simulink model "Rule_based_stop_if_likely_collision_simulink_joystick_from_odom"  (R2023a)
settings: Solver=FixedStepAuto  StartTime=0.0  StopTime=inf  RelTol=1e-3
model workspace (MAT data in the model file):
  SL_ROS_VariableLengthArrays_MaxSizes.CommonInfo.ArrayTruncateAction = 'EmitWarning'
  SL_ROS_VariableLengthArrays_MaxSizes.MsgTypeMap = containers.Map
  SL_ROS_VariableLengthArrays_MaxSizes.MsgTypeMap.serialization.keys = {'sensor_msgs/LaserScan'}
  SL_ROS_VariableLengthArrays_MaxSizes.MsgTypeMap.serialization.values{1}(1).PropertyName = 'intensities'
  SL_ROS_VariableLengthArrays_MaxSizes.MsgTypeMap.serialization.values{1}(1).DataType = 'single'
  SL_ROS_VariableLengthArrays_MaxSizes.MsgTypeMap.serialization.values{1}(1).MaxLength = 360
  SL_ROS_VariableLengthArrays_MaxSizes.MsgTypeMap.serialization.values{1}(2).PropertyName = 'ranges'
  SL_ROS_VariableLengthArrays_MaxSizes.MsgTypeMap.serialization.values{1}(2).DataType = 'single'
  SL_ROS_VariableLengthArrays_MaxSizes.MsgTypeMap.serialization.values{1}(2).MaxLength = 360
  SL_ROS_VariableLengthArrays_MaxSizes.MsgTypeMap.serialization.uniformity = 0
  SL_ROS_VariableLengthArrays_MaxSizes.MsgTypeMap.serialization.keyType = 'char'
  SL_ROS_VariableLengthArrays_MaxSizes.MsgTypeMap.serialization.valueType = 'any'
values from neighbouring files (symbols this model uses):
  scan = lidarScan(ranges,angles)    [rule_based_obstacles_avoidance_stop_if_likely_collision.m]
undefined symbols (not defined in the file or in its folder): angular, linear
libraries: ros2lib x5, vrlib x1
settings Model: Creator=fede  LastModifiedBy=fede
settings OptimizationCC: EnhancedBackFolding=on  PassReuseOutputArgsAs=Individual arguments  ZeroExternalMemoryAtStartup=off  ZeroInternalMemoryAtStartup=off  MaxStackSize=64  OptimizeBlockOrder=speed  DifferentSizesBufferReuse=on  OptimizationCustomize=off  EfficientTunableParamExpr=on
settings DebuggingCC: ParameterTunabilityLossMsg=error
settings HardwareCC: ProdBitPerLong=64  ProdHWDeviceType=Intel->x86-64 (Linux 64)  UseEmbeddedCoderFeatures=off
settings SFSimCC: MATLABDynamicMemAlloc=off
settings RTWCC: Description=Embedded Coder  SystemTargetFile=ert.tlc  HardwareBoard=Robot Operating System 2 (ROS 2)  TLCOptions="-aInlineSetEventsForThisBaseRateFcn=TLC_FALSE -aSuppressMultiTaskScheduler=TLC_FALSE  -aRateBasedStepFcn=0"  TemplateMakefile=ert_default_tmf  Toolchain=Colcon Tools  TargetLang=C++
settings CodeAppCC: ForceParamTrailComments=on  IgnoreCustomStorageClasses=off  OperatorAnnotations=on  SimulinkDataObjDesc=on  SFDataObjDesc=on  InsertBlockDesc=on
settings ERTTargetCC: CodeInterfacePackaging=C++ class  SupportNonInlinedSFcns=on  RootIOFormat=Structure reference

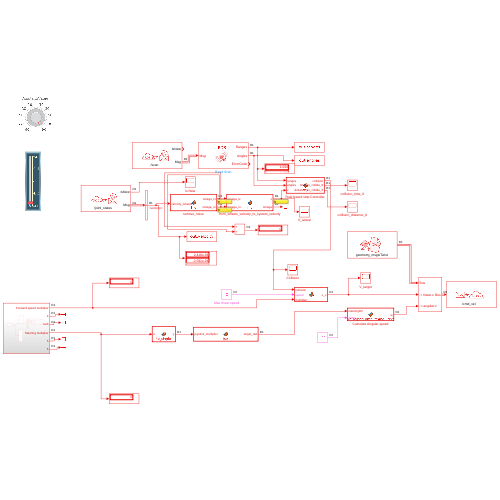
[thumbnail: Simulink's stored preview of the top-level diagram]
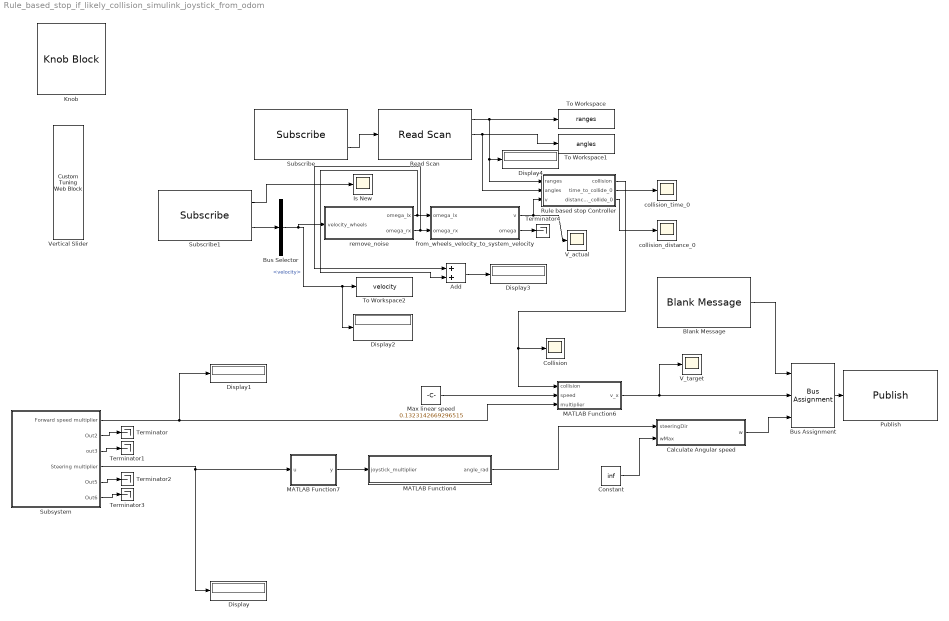
== system Rule_based_stop_if_likely_collision_simulink_joystick_from_odom ==
  Add : Sum
  Blank Message : ros2lib/Blank Message  messageClass=Message  entityType=geometry_msgs/Twist  messageType=geometry_msgs/Twist  SampleTime=0.01
  Bus Assignment : BusAssignment  AssignedSignals=linear.x,angular.z
  Bus Selector : BusSelector  OutputSignals=velocity
  Calculate Angular speed : MATLAB Function  TreatAsAtomicUnit=on
  Collision : Scope
  Constant : Constant  Value=inf
  Display{,1..4} (5 alike) : Display
  Is New : Scope
  Knob : KnobBlock  ScaleMin=-90  ScaleMax=90
  MATLAB Function4 : MATLAB Function  TreatAsAtomicUnit=on  SystemSampleTime=0.01
  MATLAB Function6 : MATLAB Function  TreatAsAtomicUnit=on  SystemSampleTime=0.01
  MATLAB Function7 : MATLAB Function  TreatAsAtomicUnit=on
  Max linear speed : Constant  Value=0.1323142669296515
  Publish : ros2lib/Publish  topicSource=Select from ROS network  topic=/cmd_vel  messageType=geometry_msgs/Twist  QOSHistory=Keep last  QOSDepth=1  QOSReliability=Reliable  QOSDurability=Volatile
  Read Scan : ros2lib/Read Scan  MaximumArrayLength=180  ShowAnglesOutput=on  ShowIntensityOutput=off  ShowErrorCodeOutput=on  VariableSizeOutputs=off
  Rule based stop Controller : MATLAB Function  TreatAsAtomicUnit=on
  Subscribe : ros2lib/Subscribe  topicSource=Select from ROS network  topic=/scan  messageType=sensor_msgs/LaserScan  sampleTime=0.01  QOSHistory=Keep last  QOSDepth=1  QOSReliability=Reliable  QOSDurability=Volatile
  Subscribe1 : ros2lib/Subscribe  topicSource=Select from ROS network  topic=/joint_states  messageType=sensor_msgs/JointState  sampleTime=0.01  QOSHistory=Keep last  QOSDepth=1  QOSReliability=Reliable  QOSDurability=Volatile
  Subsystem : Subsystem
  Terminator{,1..4} (5 alike) : Terminator
  To Workspace : ToWorkspace  VariableName=ranges  SaveFormat=Timeseries  SampleTime=-1
  To Workspace1 : ToWorkspace  VariableName=angles  SaveFormat=Timeseries  SampleTime=-1
  To Workspace2 : ToWorkspace  VariableName=velocity  SaveFormat=Timeseries  SampleTime=-1
  V_actual : Scope
  V_target : Scope
  Vertical Slider : CustomTuningWebBlock  LabelPosition=Hide  ShowInitialText=on  Configuration="{\"components\":[{\"name\":\"LinearScaleComponent\",\"settings\":{\"bounds\":{\"max\":2,\"min\":0,\"tickInterval\":\"auto\"},\"internalTickHeightScaleFactor\":0.5,\"labelColor\":[255,255,200],\"labelFont\":{\"font\":\"Arial\",\"fontSize\":12},\"labelOffset\":0.05,\"labelTransparency\":1,\"needleImage\":{\"size\":[596,842],\"src\":\"data:image\\/svg+xml;base64,PD94bWwgdmVyc2lvbj0iMS4wIiBlbmNvZGluZz0idXRmLTgiPz4NCjwhLS0gR2VuZXJhdG9yOiBBZG9iZSBJbGx1c3RyYXRvciAyNS4wLjAsIFNWRyBFeHBvcnQgUGx1Zy1JbiAuIFNWRyBWZXJzaW9uOiA2LjAwIEJ1aWxkIDApICAtLT4NCjxzdmcgdmVyc2lvbj0iMS4xIg0KCSBpZD0ic3ZnOCIgeG1sbnM6Y2M9Imh0dHA6Ly9jcmVhdGl2ZWNvbW1vbnMub3JnL25zIyIgeG1sbnM6ZGM9Imh0dHA6Ly9wdXJsLm9yZy9kYy9lbGVtZW50cy8xLjEvIiB4bWxuczppbmtzY2FwZT0iaHR0cDovL3d3dy5pbmtzY2FwZS5vcmcvbmFtZXNw ...(+2420 chars)\",\"srcOrientation\":\"horizontal\"},\"needleOffset\":[0.0642123287671233,-0.8044596912521441],\"needleSize\":{\"height\":0.07668067226890757,\"width\":0.4337797619047619},\"position\":[0.03623949579831933,0.2829861111111111,0.6088789682539683,0.9196428571428571],\"referencePoint\":\"auto\",\"scaleColors\":[],\"scaleColorsSize\":0.2,\"scaleDirection\":\"BT\",\"showLabels\":1,\"showMinorTicks\":0,\"showSpanLine\":1,\"showTicks\":1,\"tickColor\":[252,252,197],\"tickTransparency\":1,\"valueBarColor\":[0,114,189],\"valueBarOffset\":-0.27,\"valueBarSize\":0.1,\"valueBarTransparency\":1}},{\"name\":\"BackgroundImageComponent\",\"settings\":{\"image\":{\"size\":[380,101],\"src\":\"data:image\\/svg+xml;base64,PHN2ZyB4bWxucz0iaHR0cDovL3d3dy53My5vcmcvMjAwMC9zdmciIHhtbG5zOnhsaW5rPSJodHRwOi8vd3d3LnczLm9yZy8xOTk5L3hsaW5rIiB2aWV3Qm94PSIwIDAgMzgwIDEwMSI+PGRlZnM+PHN0eWxlPi5jbHMtMXtmaWxsOiMwMDJiNDI7fS5jbHMtMntmaWxsOiM0MjcwODI7fS5jbHMtM3tmaWxsOnVybCgjcmFkaWFsLWdyYWRpZW50KTt9LmNscy00e2ZpbGw6I2M4YzhjODtzdHJva2U6IzAwMDt9PC9zdHlsZT48cmFkaWFsR3JhZGllbnQgaWQ9InJhZGlhbC1ncmFkaWVudCIgY3g9IjE5MCIgY3k9IjUwLjUiIHI9IjI2OS4yMSIgZ3JhZGllbnRVbml0cz0idXNlclNwYWNlT25Vc2UiPjxzdG9wIG9mZnNldD0iMC4wMSIgc3RvcC1jb2xvcj0iIzNlNGY1OCIvPjxzdG9wIG9mZnNldD0iMC4wNiIgc3RvcC1jb2xvcj0iIzQ0NTc2MSIvPjxzdG9wIG9mZnNldD0iMC4xNSIgc3RvcC1jb2xvcj0iIzU1NmE3NiIvPjxzdG9wIG9mZnNldD0iMC4yNSIgc3RvcC1jb2xvcj0iIzZkODg5NSIvPjxzdG9wIG9mZnNldD0iMC4zOCIgc3RvcC1jb2xvcj0iIzhmYjJjMyIvPjxzdG9wIG9mZnNldD0iMC41MiIgc3RvcC1jb2xvcj0iI2I2ZTRmYSIvPjxzdG9wIG9mZnNldD0iMSIgc3RvcC1jb2xvcj0iIzE1NDY1NyIvPjwvcmFkaWFsR3JhZGllbnQ+PC9kZWZzPjxnIGlkPSJmcmFtZSI+PGcgaWQ9IkxheWVyXzIiIGRhdGEtbmFtZT0iTGF5ZXIgMiI+PGcgaWQ9IkxheWVyXzEtMiIgZGF0YS1uYW1lPSJMYXllciAxLTIiPjxyZWN0IGlkPSJyZWN0MTAzNiIgY2xhc3M9ImNscy0xIiB4PSIxMSIgeT0iMTEiIHdpZHRoPSIzNTgiIGhlaWdodD0iNzkiLz48cGF0aCBpZD0icGF0aDEwMzgiIGNsYXNzPSJjbHMtMiIgZD0iTTgsOFY5M0gzNzJWOFpNMzY5LDkwSDExVjExSDM2OVoiLz48cGF0aCBpZD0icGF0aDEwNDAiIGNsYXNzPSJjbHMtMyIgZD0iTTAsMFYxMDFIMzgwVjBaTTM3Miw5M0g4VjhIMzcyWiIvPjwvZz48L2c+PC9nPjxnIGlkPSJ0cmFjayI+PHBhdGggaWQ9InJlY3QxNjExIiBjbGFzcz0iY2xzLTQiIGQ9Ik0zMy4zNywyNi41OUgzNDYuNjNjNCwwLDcuMjUsMi42LDcuMjUsNS44MWgwYzAsMy4yMS0zLjI1LDUuODItNy4yNSw1LjgySDMzLjM3Yy00LDAtNy4yNS0yLjYxLTcuMjUtNS44MmgwQzI2LjEyLDI5LjE5LDI5LjM3LDI2LjU5LDMzLjM3LDI2LjU5WiIvPjwvZz48L3N2Zz4=\",\"srcOrientation\":\"horizontal\"},\"position\":[0,0,1,1],\"scaleMode\":\"0\"}},{\"name\":\"ForegroundImageComponent\",\"settings\":{\"image\":{\"size\":[0,0],\"src\":\"default\",\"srcOrientation\":[]},\"isForeground\":1,\"position\":[0,0,1,1],\"scaleMode\":\"0\"}}],\"settings\":{\"BindingType\":\"param\",\"aspectRatio\":3.7777777777777777,\"backgroundColor\":[0,0,0,\"1\"],\"backgroundOffset\":0,\"backgroundOpacity\":1,\"fixedAspectRatio\":\"on\",\"foregroundColor\":[252,252,196],\"orientation\":\"vertical\",\"showBackgroundColor\":false,\"value\":0,\"version\":\"R2023a\"},\"type\":\"LinearGauge\"}"
  collision_distance_0 : Scope
  collision_time_0 : Scope
  from_wheels_velocity_to_system_velocity : MATLAB Function  TreatAsAtomicUnit=on  SystemSampleTime=0.01
  remove_noise : MATLAB Function  TreatAsAtomicUnit=on  SystemSampleTime=0.01
  wires:
  Subscribe/2 -> Read Scan/1
  Read Scan/2 -> To Workspace1/1, Rule based stop Controller/2(angles)
  Blank Message/1 -> Bus Assignment/1
  Bus Assignment/1 -> Publish/1
  Subsystem/3(out3) -> Terminator1/1
  Subsystem/5(Out5) -> Terminator2/1
  Subsystem/6(Out6) -> Terminator3/1
  Subsystem/2(Out2) -> Terminator/1
  MATLAB Function6/1(v_x) -> V_target/1, Bus Assignment/2
  Max linear speed/1 -> MATLAB Function6/2(speed)
  MATLAB Function7/1(y) -> MATLAB Function4/1(joystick_multiplier)
  Calculate Angular speed/1(w) -> Bus Assignment/3
  Constant/1 -> Calculate Angular speed/2(wMax)
  Bus Selector/1 -> remove_noise/1(velocity_wheels), To Workspace2/1, Display2/1  "<velocity>"
  Rule based stop Controller/1(collision) -> Collision/1, MATLAB Function6/1(collision)
  MATLAB Function4/1(angle_rad) -> Calculate Angular speed/1(steeringDir)
  Subsystem/4(Steering multiplier) -> Display/1, MATLAB Function7/1(u)
  Subsystem/1(Forward speed multiplier) -> Display1/1, MATLAB Function6/3(multiplier)
  Subscribe1/2 -> Bus Selector/1
  Subscribe1/1 -> Is New/1
  from_wheels_velocity_to_system_velocity/1(v) -> Rule based stop Controller/3(v), V_actual/1
  from_wheels_velocity_to_system_velocity/2(omega) -> Terminator4/1
  remove_noise/1(omega_lx) -> Add/2, from_wheels_velocity_to_system_velocity/1(omega_lx)
  remove_noise/2(omega_rx) -> Add/1, from_wheels_velocity_to_system_velocity/2(omega_rx)
  Add/1 -> Display3/1
  Read Scan/1 -> To Workspace/1, Display4/1, Rule based stop Controller/1(ranges)
  Rule based stop Controller/2(time_to_collide_0) -> collision_time_0/1
  Rule based stop Controller/3(distance_to_collide_0) -> collision_distance_0/1

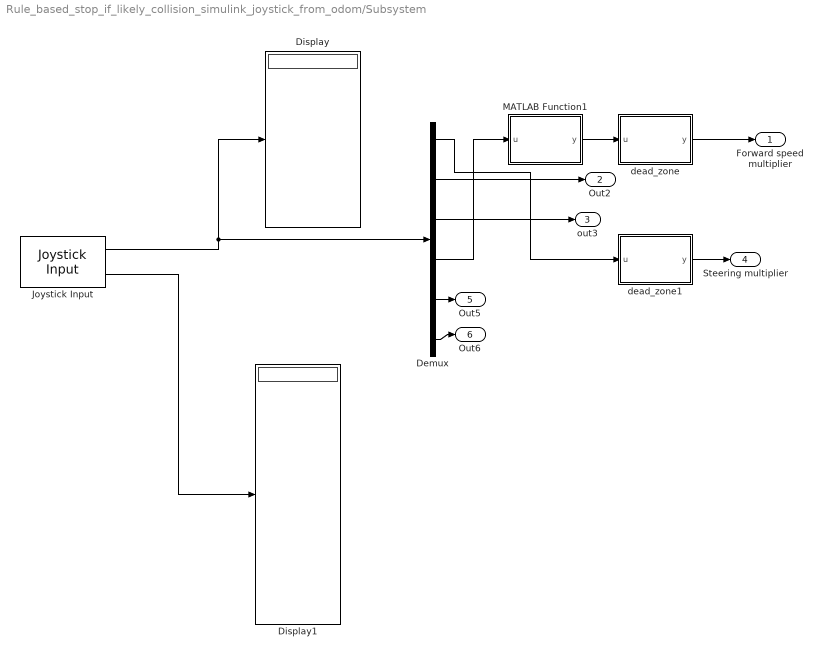
== system Rule_based_stop_if_likely_collision_simulink_joystick_from_odom/Subsystem ==
  Demux : Demux  Outputs=6
  Display : Display
  Display1 : Display
  Joystick Input : vrlib/Joystick Input  joyid=1  adjustports=on  forcefeed=off
  MATLAB Function1 : MATLAB Function  TreatAsAtomicUnit=on
  dead_zone : MATLAB Function  TreatAsAtomicUnit=on
  dead_zone1 : MATLAB Function  TreatAsAtomicUnit=on
  Forward speed multiplier : Outport
  Out2 : Outport  Port=2
  out3 : Outport  Port=3
  Steering multiplier : Outport  Port=4
  Out5 : Outport  Port=5
  Out6 : Outport  Port=6
  wires:
  Demux/2 -> Out2/1
  Demux/6 -> Out6/1
  Joystick Input/2 -> Display1/1
  Demux/5 -> Out5/1
  Joystick Input/1 -> Display/1, Demux/1
  Demux/3 -> out3/1
  MATLAB Function1/1(y) -> dead_zone/1(u)
  dead_zone/1(y) -> Forward speed multiplier/1
  dead_zone1/1(y) -> Steering multiplier/1
  Demux/4 -> MATLAB Function1/1(u)
  Demux/1 -> dead_zone1/1(u)

== matlab function Rule_based_stop_if_likely_collision_simulink_joystick_from_odom/Subsystem/MATLAB Function1 ==
  data: u input; y output
function y = fcn(u)
centered_value = u + 0.3616;

output_end = 1;
output_start = -1;
input_end = 0.7549;
input_start = -0.6384;

slope = (output_end - output_start) / (input_end - input_start);

y = -1*(output_start + slope * (centered_value - input_start));

== matlab function Rule_based_stop_if_likely_collision_simulink_joystick_from_odom/Rule based stop Controller ==
  data: ranges input; collision output; angles input; v input; time_to_collide_0 output; distance_to_collide_0 output
function [collision, time_to_collide_0, distance_to_collide_0] = fcn(ranges, angles, v)

    %Ranges, angles -> from lidar
    % v -> current wheelchair linear speed
    %Config parameters
    semi_amplitude_collision_cone_degree = 4;
    t_second_reaction_time_threshold = 3;
    %--------------

    collision_cone_rad = deg2rad(semi_amplitude_collision_cone_degree);

    %Get matrix with all 0s except 1 for elements related to the collision cone
    collision_cone_matrix_indexes = angles >= -collision_cone_rad & angles <= collision_cone_rad;
    
    %Get distances of points detected by lidar in collision cone amplitude
    collision_cone_distances = ranges(collision_cone_matrix_indexes);

    distance_to_collide_0 = collision_cone_distances(4);
    time_to_collide_0 = collision_cone_distances(4)/v;
    %Set the variable to a non-zero value if there is at least one point that is probable to collide
    %find(X,n) returns the first n indices corresponding to the nonzero elements in X.

    % Pseudo-code
    % for elem in collision_cone_distances:
    %     t = elem/v
    %     if(t<t_second_reaction_time_threshold)
    %         collision!
    if( ( v == 0 ) || ( isempty( find(collision_cone_distances/v <= t_second_reaction_time_threshold, 1) ) ) )

        collision = 0;

    elseif (v < 0) 
        % For now we decide not to take action, i.e when driving backwars
        % there is not safety system on
        collision = 0;

    else

        collision = 1;

    end

== matlab function Rule_based_stop_if_likely_collision_simulink_joystick_from_odom/Subsystem/dead_zone ==
  data: u input; y output
function y = dead_zone(u)

if(abs(u) < 0.1)
    u=0;
end

y = u;

== matlab function Rule_based_stop_if_likely_collision_simulink_joystick_from_odom/Subsystem/dead_zone1 ==
  data: u input; y output
function y = dead_zone(u)

if(abs(u) < 0.1)
    u=0;
end

y = u;

== matlab function Rule_based_stop_if_likely_collision_simulink_joystick_from_odom/from_wheels_velocity_to_system_velocity ==
  data: omega_lx input; v output double; omega output; omega_rx input
function [v,omega] = fnc(omega_lx, omega_rx)

noise_threshold = 10^-3; % obtained observing noise values

%Params
r = 0.033; %wheels radius [m]
L_r = 0.16; %distance between wheels [m]
%%%%%%%%%%%%%%%%%%%%%
v = (r / 2) * (omega_rx + omega_lx); % [m/s]

omega = (r / L_r) * (omega_rx - omega_lx); % [rad/s]

%Removing noise
if(abs(v) < noise_threshold)
    v = 0;
end

if(abs(omega) < noise_threshold)
    omega = 0;
end

== matlab function Rule_based_stop_if_likely_collision_simulink_joystick_from_odom/MATLAB Function4 ==
  data: joystick_multiplier input; angle_rad output double
function angle_rad = fcn(joystick_multiplier)

angle_rad = double(-pi/4 * joystick_multiplier);

== matlab function Rule_based_stop_if_likely_collision_simulink_joystick_from_odom/remove_noise ==
  data: velocity_wheels input; omega_lx output double; omega_rx output
function [omega_lx,omega_rx] = fnc(velocity_wheels)

noise_threshold = 10^-3; % obtained observing noise values

if(abs(velocity_wheels(1)) < noise_threshold)
    omega_lx = 0;
else
    % omega_lx = round(velocity_wheels(1)*100)/100;
    omega_lx = velocity_wheels(1);
end

if(abs(velocity_wheels(2)) < noise_threshold)
    omega_rx = 0;
else
    % omega_rx = round(velocity_wheels(2)*100/100);
    omega_rx = velocity_wheels(2);
end

== matlab function Rule_based_stop_if_likely_collision_simulink_joystick_from_odom/MATLAB Function6 ==
  data: collision input; speed input; v_x output; multiplier input
function v_x = fcn(collision, speed, multiplier)

    if(collision == 1)
    
        v_x = 0;
    
    else
        
        v_x = speed * multiplier;
    
    end

== matlab function Rule_based_stop_if_likely_collision_simulink_joystick_from_odom/MATLAB Function7 ==
  data: u input; y output
function y = to_single(u)

y = single(u);

== matlab function Rule_based_stop_if_likely_collision_simulink_joystick_from_odom/Calculate Angular speed ==
  data: steeringDir input; w output; wMax input
function w = exampleHelperComputeAngularVelocity(steeringDir, wMax)
%EXAMPLEHELPERCOMPUTEANGULARVELOCITY Compute angular velocity
%   W = exampleHelperComputeAngularVelocity(STEERINGDIR)
%   returns the angular velocity W for a differential drive robot in radians
%   per second for a given steering direction STEERINGDIR in the robot's
%   coordinate frame in radians.
%
%   W = exampleHelperComputeAngularVelocity(STEERINGDIR, WMAX)
%   returns the angular velocity W for a differential drive robot in radians
%   per second for a given steering direction STEERINGDIR in the robot's
%   coordinate frame in radians and maximum angular velocity WMAX in
%   radians per second. The output angular velocity is saturated based on
%   the WMAX.
%
%   Example:
%       
%       w = exampleHelperComputeAngularVelocity(0.2, 1);

% Copyright 2015 The MathWorks, Inc.

%#codegen
%#ok<*EMCA>

% Allow variable input arguments
if nargin == 1   
    wMax = inf;
end

validateattributes(steeringDir, {'double'},{'real'},...
    'exampleHelperComputeAngularVelocity', 'STEERINGDIR', 1);
validateattributes(wMax, {'double'},{'real', 'positive'},...
    'exampleHelperComputeAngularVelocity', 'WMAX', 2);

% Computing in robot's coordinate frame
curPose = [0 0 0];

% The following computation is similar to robotics.PurePursuit
lookaheadPoint = [cos(steeringDir), sin(steeringDir)];
slope = atan2((lookaheadPoint(2) - curPose(2)), ...
    (lookaheadPoint(1) - curPose(1)));
alpha = angdiff(curPose(3), slope);

% Angular velocity command for a differential drive robot is
% equal to the desired curvature to be followed by the robot.

w = (2*sin(alpha));

% Pick a constant rotation when robot is facing in the opposite
% direction of the path
if abs(abs(alpha) - pi) < 1e-12
    w = sign(w)*1;
end

if abs(w) > wMax
    w = sign(w)*wMax;
end

end
